simulink model "fangzheng_run"  (R2024b)
settings: Solver=ode5  StartTime=0.0  StopTime=600  FixedStep=0.05  RelTol=1e-3
values from neighbouring files (symbols this model uses):
  Ini_Omega = 1.59    [fangzheng.m]    (also in setup_sim.m)
  J_total = Jr + (ng^2) * Jg    (= 464744.67254)    [fangzheng.m]    (also in setup_sim.m = 504744.67254)
  R = 20    [fangzheng.m]    (also in setup_sim.m)
  rho = 1.225    [fangzheng.m]    (also in setup_sim.m)
settings Model: Creator=ADMIN  LastModifiedBy=elaina
settings DataIOCC: ReturnWorkspaceOutputs=off

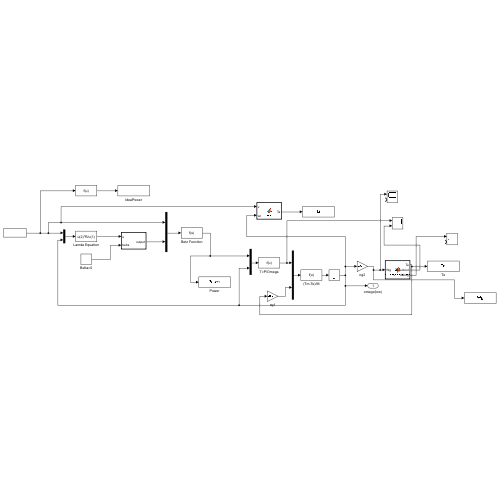
[thumbnail: Simulink's stored preview of the top-level diagram]
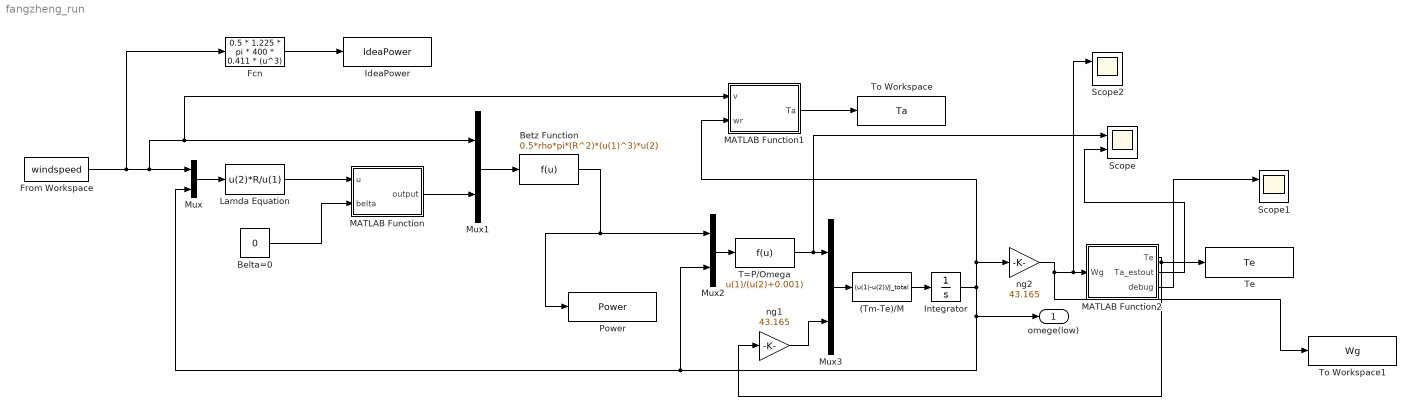
== system fangzheng_run ==
  (Tm-Te)/M : Fcn  Expr=(u(1)-u(2))/J_total
  Belta=0 : Constant  Value=0
  Betz Function : Fcn  Expr=0.5*rho*pi*(R^2)*(u(1)^3)*u(2)
  Fcn : Fcn  Expr=0.5 * 1.225 * pi * 400 * 0.411 * (u^3)
  From Workspace : FromWorkspace  VariableName=windspeed
  IdeaPower : ToWorkspace  VariableName=IdeaPower  SaveFormat=Timeseries  SampleTime=-1
  Integrator : Integrator  InitialCondition=Ini_Omega
  Lamda Equation : Fcn  Expr=u(2)*R/u(1)
  MATLAB Function : MATLAB Function  TreatAsAtomicUnit=on
  MATLAB Function1 : MATLAB Function  TreatAsAtomicUnit=on
  MATLAB Function2 : MATLAB Function  TreatAsAtomicUnit=on  SystemSampleTime=0.05
  Mux{,1..3} (4 alike) : Mux  Inputs=2
  Power : ToWorkspace  VariableName=Power  SaveFormat=Timeseries  SampleTime=-1
  Scope : Scope  NumInputPorts=2
  Scope1 : Scope  NumInputPorts=2
  Scope2 : Scope  NumInputPorts=2
  T=P/Omega : Fcn  Expr=u(1)/(u(2)+0.001)
  Te : ToWorkspace  VariableName=Te  SampleTime=-1
  To Workspace : ToWorkspace  VariableName=Ta  SaveFormat=Timeseries  SampleTime=-1
  To Workspace1 : ToWorkspace  VariableName=Wg  SaveFormat=Timeseries  SampleTime=-1
  ng1 : Gain  Gain=43.165
  ng2 : Gain  Gain=43.165
  omege(low) : Outport
  wires:
  From Workspace/1 -> Fcn/1, MATLAB Function1/1(v), Mux1/1, Mux/1
  Belta=0/1 -> MATLAB Function/2(belta)
  Mux/1 -> Lamda Equation/1
  Lamda Equation/1 -> MATLAB Function/1(u)
  MATLAB Function/1(output) -> Mux1/2
  Mux1/1 -> Betz Function/1
  Betz Function/1 -> Power/1, Mux2/1
  Mux2/1 -> T=P/Omega/1
  Mux3/1 -> (Tm-Te)/M/1
  (Tm-Te)/M/1 -> Integrator/1
  T=P/Omega/1 -> Scope/1, Mux3/1
  ng2/1 -> To Workspace1/1, Scope2/1, MATLAB Function2/1(Wg)
  MATLAB Function2/1(Te) -> ng1/1, Te/1
  Fcn/1 -> IdeaPower/1
  Integrator/1 -> MATLAB Function1/2(wr), ng2/1, Mux2/2, Mux/2, omege(low)/1
  MATLAB Function1/1(Ta) -> To Workspace/1
  ng1/1 -> Mux3/2
  MATLAB Function2/2(Ta_estout) -> Scope/2
  MATLAB Function2/3(debug) -> Scope1/1

== matlab function fangzheng_run/MATLAB Function1 ==
  data: v input; Ta output; wr input
function Ta = fcn(v, wr)
% 这是一个计算风机气动转矩的模块
% 输入 v : 实时风速 (m/s)
% 输入 wr: 低速轴风轮转速 (rad/s)
% 输出 Ta: 气动转矩 (Nm)

% 1. 定义 600kW 风机的固有参数
R = 20;           % 风轮半径 (m)
rho = 1.225;      % 空气密度 (kg/m^3)
beta = 0;         % 桨距角 (MPPT阶段通常恒为0度)

% 2. 容错处理：防止仿真初期转速或风速为0导致除以零报错
if v < 0.1
    v = 0.1;
end
if wr < 0.1
    wr = 0.1;
end

% 3. 计算叶尖速比 Lambda
lambda = (wr * R) / v;

% 4. 计算风能利用系数 Cp
% （这里使用的是风电领域最经典通用的 Cp 解析函数，你也可以替换成你课件上特定的公式）
lambda_i = 1 / (1 / (lambda + 0.08 * beta) - 0.035 / (beta^3 + 1));
Cp = 0.5176 * (116 / lambda_i - 0.4 * beta - 5) * exp(-21 / lambda_i) + 0.0068 * lambda;

% 限制 Cp 的下限，防止出现发电机倒拖风轮的负功率现象
if Cp < 0
    Cp = 0;
end

% 5. 计算气动功率 Pa 和 气动转矩 Ta
Pa = 0.5 * rho * pi * R^2 * v^3 * Cp;
Ta = Pa / wr;

end

== matlab function fangzheng_run/MATLAB Function ==
  data: u input; output output; belta input
function output = fcn(u, belta)
    % u 对应叶尖速比 lambda，belta 对应桨距角 beta
    
    % 直接计算 1/A 的整体值，命名为 invA
    invA = 1 / (u + 0.08 * belta) - 0.035;
    
    % 注意：指数必须使用 exp() 函数
    C_p = 0.5 * (116 * invA - 0.4 * belta - 5) * exp(-21 * invA);
    
    % 防止物理上不可能的负风能捕获
    if C_p < 0
        C_p = 0;
    end
    
    output = C_p;
end

== matlab function fangzheng_run/MATLAB Function2 ==
  data: Wg input; Te output; Ta_estout output; debug output
function [Te, Ta_estout,debug] = fcn_instant_custom(Wg)
    % 修正版：考虑齿轮箱变比的 Ta 观测器
    % Wg: 发电机转速 (rad/s)
    % Te: 发电机电磁转矩 (N·m)
    
    persistent prev_Wg prev_Te Ta_est
    dt = 0.05; 
    i_ratio = 43; % 减速比
    
    % --- 1. 参数定义 ---
    K_opt = 0.0626;    
    % 重要：如果 504740 是风轮侧惯量，折算到发电机侧需除以 i^2
    J_LSS = 504740; 
    J_HSS = J_LSS / (i_ratio^2); % 折算后的等效惯量
    
    L_obs = 0.5;       
    W_gbgn = 56;       
    
    if isempty(prev_Wg)
        prev_Wg = Wg;
        prev_Te = 0;
        Ta_est = K_opt * (Wg^2); 
    end
    
    % --- 2. 机械转矩 (Ta) 观测器 (在发电机轴侧进行计算) ---
    % 此时观测到的是“折算到高速轴的机械转矩”
    d_Wg = (Wg - prev_Wg) / dt;
    Ta_HSS_instant = J_HSS * d_Wg + prev_Te; 
    Ta_est = (1 - L_obs) * Ta_est + L_obs * Ta_HSS_instant;
    
    % --- 3. 计算最优转矩与补偿 ---
    Te_ideal = K_opt * (Wg^2);
    delta_Wg = Wg - prev_Wg;
    
    if Wg < W_gbgn
        Te_raw = 0;
    else
        if delta_Wg > 0
            % 【上升阶段】
            K_acc_gain = 1.0; % 既然有了准确的观测，可以适当调大补偿
            % 如果 Ta_est > Te_ideal，说明风能输入大于当前发电机吸收，支持加速
            Te_raw = Te_ideal - K_acc_gain * (Ta_est - Te_ideal);
        else
            % 【下降阶段】
            fall_rate = 0.95; 
            Te_raw = prev_Te * fall_rate + Te_ideal * (1 - fall_rate);
        end
    end
    
    % --- 4. 限幅与更新 ---
    Te = max(0, min(Te_raw, 12000));
    
    % 如果你想输出风轮端的实际转矩 Ta，则需要乘以 i_ratio
    Ta_estout = Ta_est * i_ratio; 
    
    prev_Wg = Wg;
    prev_Te = Te;
    debug=Ta_est-Te_ideal;
end
